simulink model "Know"  (R2023a)
settings: Solver=VariableStepAuto  StartTime=0.0  StopTime=0.02  RelTol=1e-3
settings Model: Creator=vande  LastModifiedBy=vande

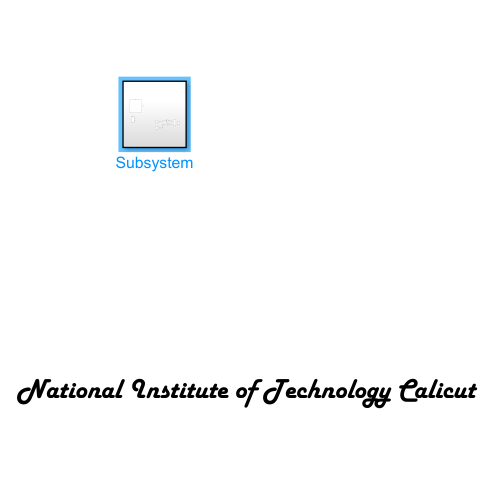
[thumbnail: Simulink's stored preview of the top-level diagram]
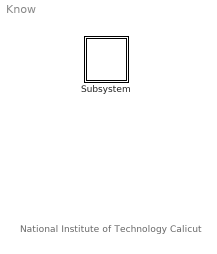
== system Know ==
  note: National Institute of Technology Calicut
  Subsystem : Subsystem

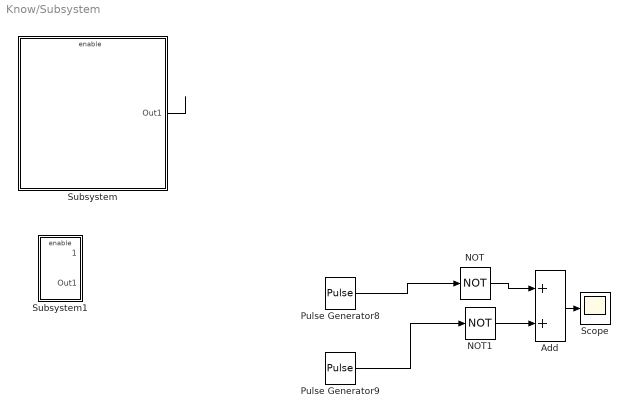
== system Know/Subsystem ==
  Add : Sum
  NOT : Logic  Operator=NOT  IconShape=distinctive  AllPortsSameDT=off  OutDataTypeStr=boolean
  NOT1 : Logic  Operator=NOT  IconShape=distinctive  AllPortsSameDT=off  OutDataTypeStr=boolean
  Pulse Generator8 : DiscretePulseGenerator  PulseType=Time based  Period=0.02  PulseWidth=(8/14)*100
  Pulse Generator9 : DiscretePulseGenerator  PulseType=Time based  Period=0.02  PulseWidth=(1/14)*100  PhaseDelay=(13/14)*0.02
  Scope : Scope
  Subsystem : Subsystem
  Subsystem1 : Subsystem
  wires:
  Subsystem/1(Out1) -> ?
  Add/1 -> Scope/1
  NOT1/1 -> Add/2
  NOT/1 -> Add/1
  Pulse Generator8/1 -> NOT/1
  Pulse Generator9/1 -> NOT1/1

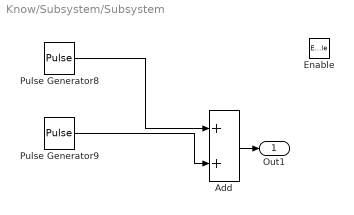
== system Know/Subsystem/Subsystem ==
  Enable : EnablePort
  Add : Sum
  Pulse Generator8 : DiscretePulseGenerator  PulseType=Time based  Period=0.02  PulseWidth=(8/14)*100
  Pulse Generator9 : DiscretePulseGenerator  PulseType=Time based  Period=0.02  PulseWidth=(1/14)*100  PhaseDelay=(13/14)*0.02
  Out1 : Outport
  wires:
  Pulse Generator9/1 -> Add/2
  Pulse Generator8/1 -> Add/1
  Add/1 -> Out1/1

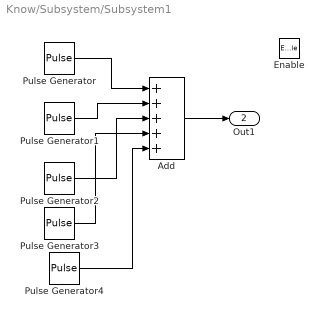
== system Know/Subsystem/Subsystem1 ==
  Enable : EnablePort
  Add : Sum  Inputs=+++++
  Pulse Generator : DiscretePulseGenerator  PulseType=Time based  Period=0.02  PulseWidth=(1/14)*100  PhaseDelay=(1/14)*0.02
  Pulse Generator1 : DiscretePulseGenerator  PulseType=Time based  Period=0.02  PulseWidth=(1/14)*100  PhaseDelay=(3/14)*0.02
  Pulse Generator2 : DiscretePulseGenerator  PulseType=Time based  Period=0.02  PulseWidth=(1/14)*100  PhaseDelay=(5/14)*0.02
  Pulse Generator3 : DiscretePulseGenerator  PulseType=Time based  Period=0.02  PulseWidth=(1/14)*100  PhaseDelay=(9/14)*0.02
  Pulse Generator4 : DiscretePulseGenerator  PulseType=Time based  Period=0.02  PulseWidth=(1/14)*100  PhaseDelay=(11/14)*0.02
  Out1 : Outport  Port=2
  wires:
  Pulse Generator3/1 -> Add/4
  Pulse Generator2/1 -> Add/3
  Pulse Generator4/1 -> Add/5
  Pulse Generator/1 -> Add/1
  Pulse Generator1/1 -> Add/2
  Add/1 -> Out1/1
